simulink model "suspension"  (R2026a)
settings: Solver=VariableStepAuto
values from neighbouring files (symbols this model uses):
  bd = 2.5e3    (= 2500)    [suspensionsystemdata.m]
  ks = 20e3    (= 20000)    [suspensionsystemdata.m]
  kt = 250e3    (= 250000)    [suspensionsystemdata.m]
  ms = 400    [suspensionsystemdata.m]
  mu = 50    [suspensionsystemdata.m]
settings Model: Creator=suria  LastModifiedBy=suria

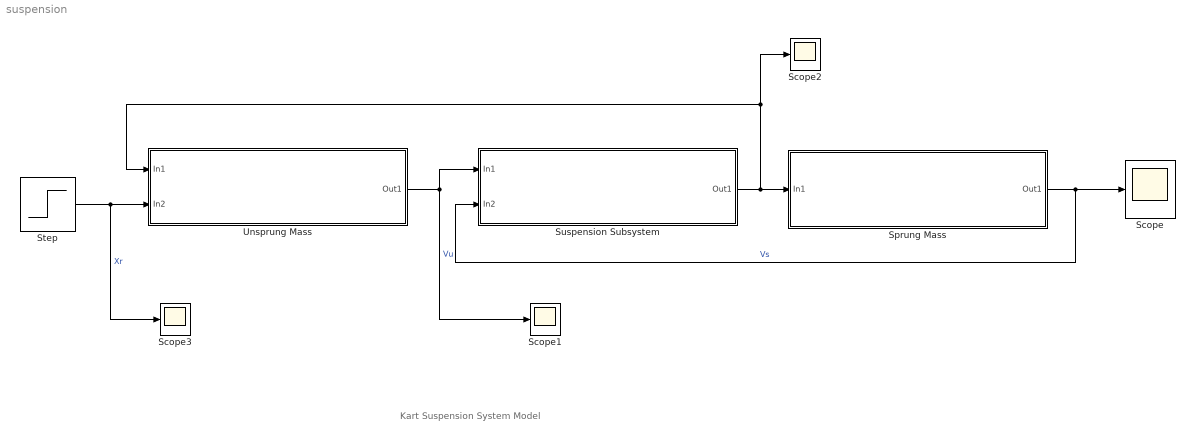
== system suspension ==
  note: Kart Suspension System Model
  Scope{,1..3} (4 alike) : Scope
      Scope settings: ActiveDisplayYMinimum=-0.28459728958821046  ActiveDisplayYMaximum=0.94805250277469655
      Scope1 settings: ActiveDisplayYMinimum=-1.8153464239367765  ActiveDisplayYMaximum=4.9638018128415569
      Scope2 settings: ActiveDisplayYMinimum=-4151.0914454096092  ActiveDisplayYMaximum=7994.6202847229224  DataLoggingVariableName=ScopeData2
      Scope3 settings: ActiveDisplayYMinimum=-0.11780615783966328  ActiveDisplayYMaximum=0.30232982481872128  DataLoggingVariableName=ScopeData4
  Sprung Mass : Subsystem
  Step : Step  FinalValue=0.1  SampleTime=0
  Suspension Subsystem : Subsystem
  Unsprung Mass : Subsystem
  wires:
  Step/1 -> Scope3/1, Unsprung Mass/2(In2)  "Xr"
  Unsprung Mass/1(Out1) -> Suspension Subsystem/1(In1), Scope1/1  "Vu"
  Sprung Mass/1(Out1) -> Suspension Subsystem/2(In2), Scope/1  "Vs"
  Suspension Subsystem/1(Out1) -> Sprung Mass/1(In1), Scope2/1, Unsprung Mass/1(In1)

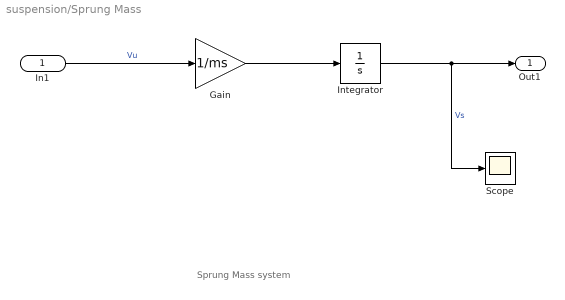
== system suspension/Sprung Mass ==
  note: Sprung Mass system
  In1 : Inport
  Gain : Gain  Gain=1/ms
  Integrator : Integrator
  Scope : Scope
      settings: ActiveDisplayYMinimum=-1  ActiveDisplayYMaximum=1  DataLoggingVariableName=ScopeData6
  Out1 : Outport
  wires:
  In1/1 -> Gain/1  "Vu"
  Gain/1 -> Integrator/1
  Integrator/1 -> Scope/1, Out1/1  "Vs"

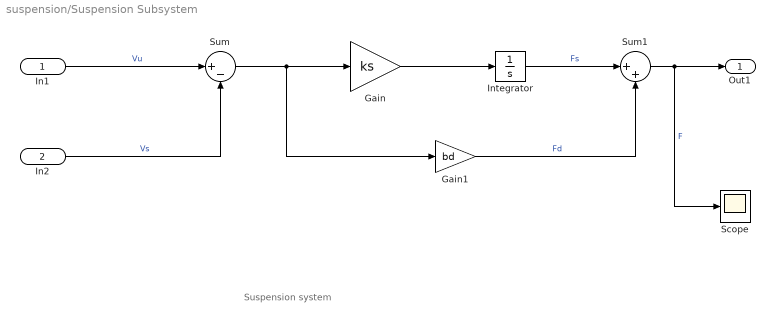
== system suspension/Suspension Subsystem ==
  note: Suspension system
  In1 : Inport
  In2 : Inport  Port=2
  Gain : Gain  Gain=ks
  Gain1 : Gain  Gain=bd
  Integrator : Integrator
  Scope : Scope
      settings: ActiveDisplayYMinimum=-1  ActiveDisplayYMaximum=1  DataLoggingVariableName=ScopeData5
  Sum : Sum  Inputs=|+-
  Sum1 : Sum  Inputs=|++
  Out1 : Outport
  wires:
  In1/1 -> Sum/1  "Vu"
  Sum/1 -> Gain1/1, Gain/1
  Gain/1 -> Integrator/1
  Integrator/1 -> Sum1/1  "Fs"
  Sum1/1 -> Scope/1, Out1/1  "F"
  In2/1 -> Sum/2  "Vs"
  Gain1/1 -> Sum1/2  "Fd"

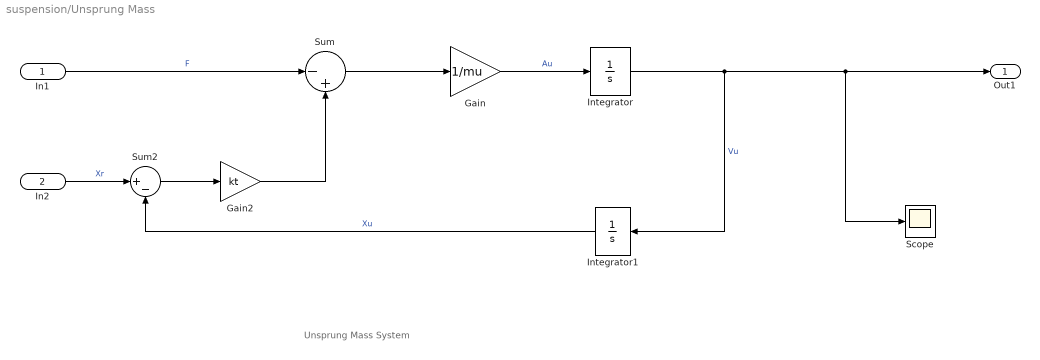
== system suspension/Unsprung Mass ==
  note: Unsprung Mass System
  In1 : Inport
  In2 : Inport  Port=2
  Gain : Gain  Gain=1/mu
  Gain2 : Gain  Gain=kt
  Integrator : Integrator
  Integrator1 : Integrator
  Scope : Scope
      settings: ActiveDisplayYMinimum=-1.4663343582038748  ActiveDisplayYMaximum=3.9220086561402172  DataLoggingVariableName=ScopeData3
  Sum : Sum  Inputs=|-+
  Sum2 : Sum  Inputs=|+-
  Out1 : Outport
  wires:
  In1/1 -> Sum/1  "F"
  Sum/1 -> Gain/1
  Gain/1 -> Integrator/1  "Au"
  Integrator/1 -> Integrator1/1, Scope/1, Out1/1  "Vu"
  In2/1 -> Sum2/1  "Xr"
  Gain2/1 -> Sum/2
  Integrator1/1 -> Sum2/2  "Xu"
  Sum2/1 -> Gain2/1
